simulink model "DynJointCon"  (Simulink 7.6)
settings: Solver=ode45  StartTime=0.0  StopTime=10.0  RelTol=1e-3
InitFcn:
  | eval('Config')
values from neighbouring files (symbols this model uses):
  a2 = 0    [Config.m]    (also in CtrPlatformCfg.m)
  a3 = 0    [Config.m]    (also in CtrPlatformCfg.m)
  a4 = 0    [Config.m]    (also in CtrPlatformCfg.m)
  a5 = 90    [Config.m]    (also in CtrPlatformCfg.m)
  a6 = 0    [Config.m]    (also in CtrPlatformCfg.m)
  Cen = Cen(:)'    [Config.m]    (also in CtrPlatformCfg.m; DynEulerTest.m = Cen'; EfDynCAD.m = [cen1,cen2,cen3,cen4,cen5,cen6]')
  freq = tvel/radius    (= 1)    [Config.m]    (also in CtrPlatformCfg.m)
  Ie1 = in1(:)'    [Config.m]    (also in CtrPlatformCfg.m; DynEulerTest.m = in1(:); EfDynCAD.m = in1(:))
  Ie2 = in2(:)'    [Config.m]    (also in CtrPlatformCfg.m; DynEulerTest.m = in2(:); EfDynCAD.m = in2(:))
  Ie3 = in3(:)'    [Config.m]    (also in CtrPlatformCfg.m; DynEulerTest.m = in3(:); EfDynCAD.m = in3(:))
  Ie4 = in4(:)'    [Config.m]    (also in CtrPlatformCfg.m; DynEulerTest.m = in4(:); EfDynCAD.m = in4(:))
  Ie5 = in5(:)'    [Config.m]    (also in CtrPlatformCfg.m; DynEulerTest.m = in5(:); EfDynCAD.m = in5(:))
  Ie6 = in6(:)'    [Config.m]    (also in CtrPlatformCfg.m; DynEulerTest.m = in6(:); EfDynCAD.m = in6(:))
  init_Endx = gd_init(1,4)    [Config.m]    (also in CtrPlatformCfg.m)
  init_Endy = gd_init(2,4)    [Config.m]    (also in CtrPlatformCfg.m)
  init_Endz = gd_init(3,4)    [Config.m]    (also in CtrPlatformCfg.m)
  init_Rot = gd_init(1:3,1:3)    [Config.m]    (also in CtrPlatformCfg.m)
  L = [l1 l2 l3 l4 l5 l6 l7 l8 l9]    [Config.m]    (also in CtrPlatformCfg.m)
  Ma = [ma1 ma2 ma3 ma4 ma5 ma6]    [Config.m]    (also in CtrPlatformCfg.m; DynEulerTest.m = [ma1; ma2; ma3; ma4; ma5; ma6]; EfDynCAD.m = [ma1 ma2 ma3 ma4 ma5 ma6]')
  tvel = 120    [Config.m]    (also in CtrPlatformCfg.m)
undefined symbols (not defined in the file or in its folder): a1
libraries: mblibv1 x35, simulink x9
(part 2 of 2)

== matlab function Line_A2A3/Jacobian ==
  data: Theta input double; Omega input double; EndVel output double; L parameter double
function EndVel = fcn(Theta,Omega,L)
%#eml


EndVW = spat_Jacobian(L,Theta')*Omega;
gd = fwd_kin(L,Theta');
EndW = EndVW(4:6,1);
gd_pos = gd(1:3,4);
EndVel=cross(EndW,gd_pos);

== matlab function Line_XZ/Inverse Kinematic ==
  data: EndPos input double; init_Rot parameter double; theta output double; L parameter double
function theta = fcn(EndPos,init_Rot,L)
%#eml
theta =[0;0; 0; 0; 0; 0];
gd = [init_Rot,EndPos;[0 0 0],1];
[theta_total,num_total] = inv_kin(gd,L);
theta = theta_total(:,2);

== matlab function Line_XZ/Jacobian ==
  data: Omega output double; EndVel input double; Theta input double; L parameter double
function Omega = fcn(EndVel,Theta,L)
%#eml

Omega = zeros(6,1);
V = [EndVel; 0; 0; 0];   
g = fwd_kin(L,Theta');
Jb = body_Jacobian(L,Theta');
Adg_inv = double(AdjointInv(g));
Omega = double((Jb \ Adg_inv* V)')';

== matlab function Circle_A2A3/Forward ==
  data: Theta input double; EndPos output double; L parameter double
function EndPos = fcn(Theta,L)
%#eml
gd = fwd_kin(L,Theta');
EndPos = gd(1:3,4);

== matlab function Circle_A2A3/Jacobian ==
  data: Theta input double; Omega input double; EndVel output double; L parameter double
function EndVel = fcn(Theta,Omega,L)
%#eml


EndVW = spat_Jacobian(L,Theta')*Omega;
gd = fwd_kin(L,Theta');
EndW = EndVW(4:6,1);
gd_pos = gd(1:3,4);
EndVel=cross(EndW,gd_pos);

== matlab function Line_A1/Forward ==
  data: Theta input double; EndPos output double; L parameter double
function EndPos = fcn(Theta,L)
%#eml
gd = fwd_kin(L,Theta');
EndPos = gd(1:3,4);

== matlab function Line_A1/Jacobian ==
  data: Theta input double; Omega input double; EndVel output double; L parameter double
function EndVel = fcn(Theta,Omega,L)
%#eml


EndVW = spat_Jacobian(L,Theta')*Omega;
gd = fwd_kin(L,Theta');
EndW = EndVW(4:6,1);
gd_pos = gd(1:3,4);
EndVel=cross(EndW,gd_pos);
